simulink model "Assignment7"  (R2019a)
settings: Solver=VariableStepAuto  StartTime=0.0  StopTime=25  RelTol=1e-3
settings Model: Creator=Bikram Kumar De  LastModifiedBy=Bikram Kumar De

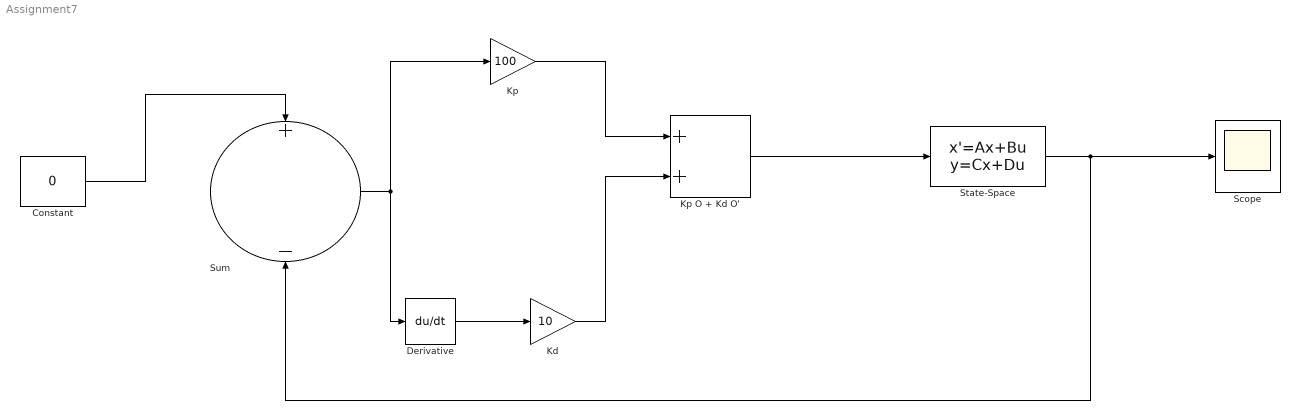
== system Assignment7 ==
  Constant : Constant  Value=0
  Derivative : Derivative
  Kd : Gain  Gain=10
  Kp : Gain  Gain=100
  Kp O + Kd O' : Sum
  Scope : Scope
  State-Space : StateSpace  A=[0 1; -1 0]  B=[0; 1]  C=[1 0]  D=[0]  InitialCondition=[1 1]
  Sum : Sum  Inputs=+-
  wires:
  Constant/1 -> Sum/1
  Kp/1 -> Kp O + Kd O'/1
  Kd/1 -> Kp O + Kd O'/2
  Derivative/1 -> Kd/1
  Sum/1 -> Kp/1, Derivative/1
  Kp O + Kd O'/1 -> State-Space/1
  State-Space/1 -> Sum/2, Scope/1
